simulink model "ATV_LAB4_SIMU_Q8"  (R2021a)
settings: Solver=VariableStepAuto  StartTime=0.0  StopTime=1800  RelTol=1e-3
settings Model: Creator=Home  LastModifiedBy=Home

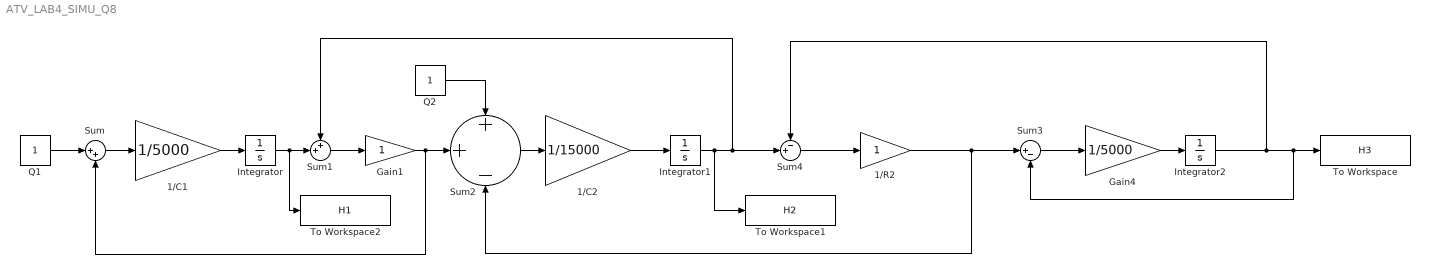
== system ATV_LAB4_SIMU_Q8 ==
  1/C1 : Gain  Gain=1/5000
  1/C2 : Gain  Gain=1/15000
  1/R2 : Gain
  Gain1 : Gain
  Gain4 : Gain  Gain=1/5000
  Integrator : Integrator
  Integrator1 : Integrator
  Integrator2 : Integrator
  Q1 : Constant
  Q2 : Constant
  Sum : Sum  Inputs=|++
  Sum1 : Sum  Inputs=++|
  Sum2 : Sum  Inputs=++-
  Sum3 : Sum  Inputs=|+-
  Sum4 : Sum  Inputs=-+|
  To Workspace : ToWorkspace  VariableName=H3  SampleTime=-1
  To Workspace1 : ToWorkspace  VariableName=H2  SampleTime=-1
  To Workspace2 : ToWorkspace  VariableName=H1  SampleTime=-1
  wires:
  Sum/1 -> 1/C1/1
  Q1/1 -> Sum/1
  1/C1/1 -> Integrator/1
  Sum1/1 -> Gain1/1
  Gain1/1 -> Sum/2, Sum2/2
  Q2/1 -> Sum2/1
  Sum2/1 -> 1/C2/1
  1/C2/1 -> Integrator1/1
  Integrator1/1 -> To Workspace1/1, Sum4/2, Sum1/1
  1/R2/1 -> Sum3/1, Sum2/3
  Sum3/1 -> Gain4/1
  Gain4/1 -> Integrator2/1
  Integrator2/1 -> Sum3/2, To Workspace/1, Sum4/1
  Integrator/1 -> To Workspace2/1, Sum1/2
  Sum4/1 -> 1/R2/1
